simulink model "ReverseParking_Model"  (Simulink 8.2)
settings: Solver=FixedStepDiscrete  SolverMode=SingleTasking  StartTime=0.0  StopTime=inf  FixedStep=1/100  RelTol=1e-3
values from neighbouring files (symbols this model uses):
  dfreq = block.DialogPrm(1).Data    [msfcn_PPS_PlotSpeed.m]    (also in msfcn_PPS_radar_graph.m)
libraries: simulink x16, simulink_extras x3
settings Model: Creator=Krzysztof  LastModifiedBy=raufk
settings DataIOCC: SaveOutput=off  SaveTime=off
settings OptimizationCC: InlineParams=on  OptimizeBlockIOStorage=off  BufferReuse=off  ExpressionFolding=off  LocalBlockOutputs=off  SimCompilerOptimization=On
settings DebuggingCC: ReadBeforeWriteMsg=DisableAll  WriteAfterWriteMsg=DisableAll  WriteAfterReadMsg=DisableAll  SolverPrmCheckMsg=none  MultiTaskDSMMsg=none  SigSpecEnsureSampleTimeMsg=none  ParameterPrecisionLossMsg=none  FrameProcessingCompatibilityMsg=error  UnknownTsInhSupMsg=none
settings ModelReferenceCC: ModelReferenceNumInstancesAllowed=Single
settings SFSimCC: SimParseCustomCode=off
settings GRTTargetCC: CodeReplacementLibrary=C89/C90 (ANSI)

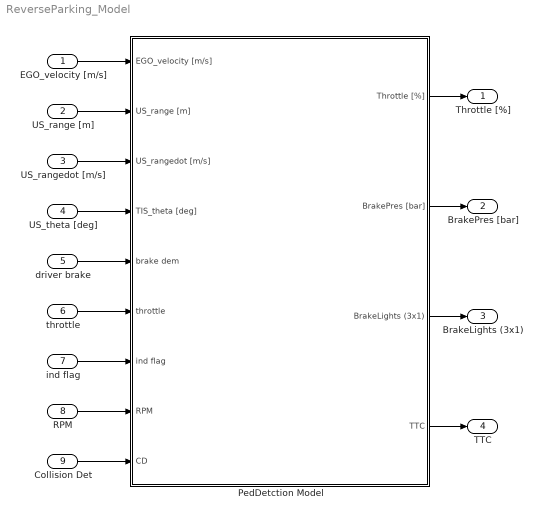
== system ReverseParking_Model ==
  EGO_velocity [m/s] : Inport
  US_range [m] : Inport  Port=2
  US_rangedot [m/s] : Inport  Port=3
  US_theta [deg] : Inport  Port=4
  driver brake : Inport  Port=5
  throttle : Inport  Port=6
  ind flag : Inport  Port=7
  RPM : Inport  Port=8
  Collision Det : Inport  Port=9
  PedDetction Model : Subsystem  mask(PPS Model){MaxSpeed=70, MaxBrakePressure=150, BrakeDelay=100, LaneWidth=3.5, USMaxRange=3, USMaxTheta=90, USfreq=20, USdet=2, Mainfreq=100}
      mask prompts: MaxSpeed "Vehicle cut-off speed [km/h]"; MaxBrakePressure "Maximum value of braking pressure available [bar]"; BrakeDelay "Braking system delay [ms]"; LaneWidth "Lane width [m]"; USMaxRange "US maximum range [m]"; USMaxTheta "US maximum theta [deg]"; USfreq "US frequency [Hz]"; USdet "Maximum Number of US Detected Objects"; Mainfreq "Compilation sheet frequency [Hz]"
      mask help: PreScan Experiment and Pedestrian Protection System parameters
      mask Help: eval('openHelp(8130)')
  Throttle [%] : Outport
  BrakePres [bar] : Outport  Port=2
  BrakeLights (3x1) : Outport  Port=3
  TTC : Outport  Port=4
  wires:
  EGO_velocity [m/s]/1 -> PedDetction Model/1(EGO_velocity [m/s])
  US_range [m]/1 -> PedDetction Model/2(US_range [m])
  US_rangedot [m/s]/1 -> PedDetction Model/3(US_rangedot [m/s])
  US_theta [deg]/1 -> PedDetction Model/4(TIS_theta [deg])
  throttle/1 -> PedDetction Model/6(throttle)
  ind flag/1 -> PedDetction Model/7(ind flag)
  PedDetction Model/1(Throttle [%]) -> Throttle [%]/1
  PedDetction Model/2(BrakePres [bar]) -> BrakePres [bar]/1
  PedDetction Model/3(BrakeLights (3x1)) -> BrakeLights (3x1)/1
  PedDetction Model/4(TTC) -> TTC/1
  driver brake/1 -> PedDetction Model/5(brake dem)
  RPM/1 -> PedDetction Model/8(RPM)
  Collision Det/1 -> PedDetction Model/9(CD)

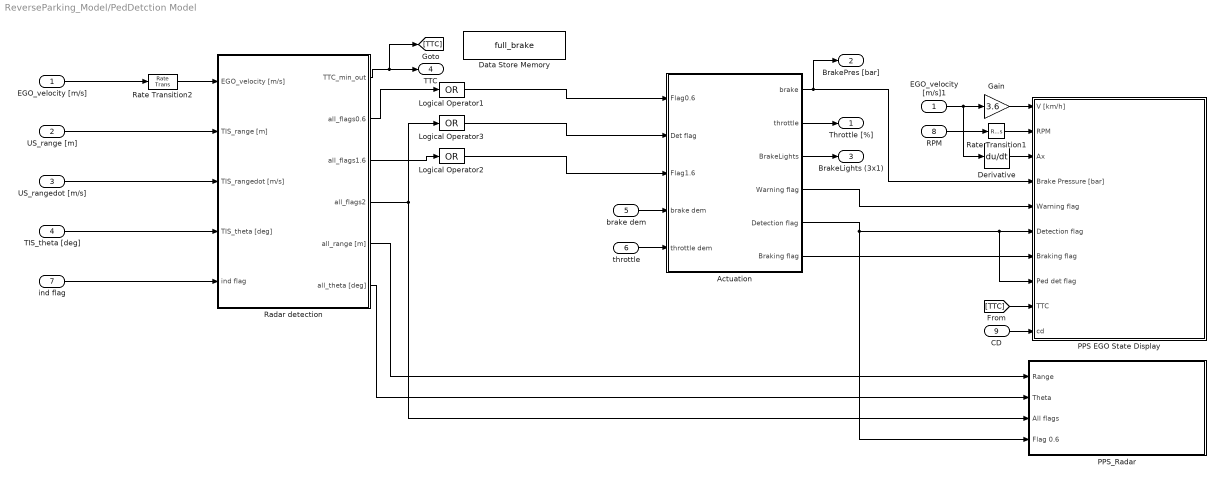
== system ReverseParking_Model/PedDetction Model ==
  EGO_velocity [m/s] : Inport
  US_range [m] : Inport  Port=2  PortDimensions=USdet  SampleTime=1/USfreq
  US_rangedot [m/s] : Inport  Port=3  PortDimensions=USdet  SampleTime=1/USfreq
  TIS_theta [deg] : Inport  Port=4  PortDimensions=USdet  SampleTime=1/USfreq
  brake dem : Inport  Port=5  SampleTime=[0,0]
  throttle : Inport  Port=6  SampleTime=[0,0]
  ind flag : Inport  Port=7  SampleTime=1/USfreq
  RPM : Inport  Port=8
  CD : Inport  Port=9
  Actuation : Subsystem
  Data Store Memory : DataStoreMemory  DataStoreName=full_brake  ReadBeforeWriteMsg=warning  WriteAfterWriteMsg=warning  WriteAfterReadMsg=warning
  Derivative : Derivative
  EGO_velocity [m/s]1 : InportShadow
  Gain : Gain  Gain=3.6
  Logical Operator1 : Logic  Operator=OR  Inputs=1  AllPortsSameDT=off  OutDataTypeStr=boolean
  Logical Operator2 : Logic  Operator=OR  Inputs=1  AllPortsSameDT=off  OutDataTypeStr=boolean
  Logical Operator3 : Logic  Operator=OR  Inputs=1  AllPortsSameDT=off  OutDataTypeStr=boolean
  PPS EGO State Display : Subsystem  StopFcn=|
      | load('VRU_DisplaySwitch');
      | load('VRU_EGO_State_Coll');
      | load('VRU_EGO_State_BrakeVel');
      | load('VRU_EGO_State_Flag06');
      | s_VRU_DisplaySwitch = VRU_DisplaySwitch(2,end);
      | s_VRU_EGO_State_Coll = VRU_EGO_State_Coll(2,end);
      | s_VRU_EGO_State_BrakeVel = VRU_EGO_State_BrakeVel(2,end);
      | s_VRU_EGO_State_Flag06 = VRU_EGO_State_Flag06(2,end);
      | 
      | if(s_VRU_DisplaySwitch)
      |   CSpanel = findobj('Tag','cs_panel');
      |   CSvalue = findobj('Tag','cs_value');
      |   
      |   if(s_VRU_EGO_State_Coll)
      |      %Collision Occured
      |      set(CSpanel, 'BorderWidth',2, 'ForegroundColor',[0 120/255 0], 'HighlightColor',[0 120/255 0], 'ShadowColor', [0 120/255 0]);
      |      set(CSvalue, 'ForegroundColor',[0 120/255 0], 'String', strcat('Speed reduction', sprintf( ' %.1f ',s_VRU_EGO_State_BrakeVel-s_VRU_EGO_State_Coll), ' km/h'));
      |      set(CSpanel, 'Visible', 'On');
      |      set(CSvalue, 'Visible', 'On');
      |   else
      |     if(s_VRU_EGO_State_Flag06)
      |         % Collision almost occur
      |         set(CSpanel, 'BorderWidth',2, 'ForegroundColor','Green', 'HighlightColor','Green', 'ShadowColor', 'Green');
      |         set(CSvalue, 'ForegroundColor','Green', 'String', 'Collision avoided');
      |         set(CSpanel, 'Visible', 'On');
      |         set(CSvalue, 'Visible', 'On');
      |      else
      |         % No risk of collision
      |         set(CSpanel, 'Visible', 'Off');
      |         set(CSvalue, 'Visible', 'Off');
      |     end
      |   end
      | 
      |   clear CSpanel CSvalue
      | end
      | 
      | PPS_Speed_Profile
      | PPS_TTC_Profile
  PPS_Radar : Subsystem
  Radar detection : Subsystem
  Rate Transition1 : RateTransition  Integrity=off  Deterministic=off  OutPortSampleTime=1/Mainfreq
  Rate Transition2 : RateTransition  Integrity=off  Deterministic=off  OutPortSampleTime=1/USfreq
  Throttle [%] : Outport
  BrakePres [bar] : Outport  Port=2
  BrakeLights (3x1) : Outport  Port=3
  TTC : Outport  Port=4
  wires:
  US_range [m]/1 -> Radar detection/2(TIS_range [m])
  US_rangedot [m/s]/1 -> Radar detection/3(TIS_rangedot [m/s])
  TIS_theta [deg]/1 -> Radar detection/4(TIS_theta [deg])
  ind flag/1 -> Radar detection/5(ind flag)
  EGO_velocity [m/s]/1 -> Rate Transition2/1
  Rate Transition2/1 -> Radar detection/1(EGO_velocity [m/s])
  throttle/1 -> Actuation/5(throttle dem)
  brake dem/1 -> Actuation/4(brake dem)
  Radar detection/1(TTC_min_out) -> TTC/1, [TTC]
  Radar detection/2(all_flags0.6) -> Logical Operator1/1
  Radar detection/4(all_flags2) -> PPS_Radar/3(All flags), Logical Operator3/1
  Radar detection/5(all_range [m]) -> PPS_Radar/1(Range)
  Radar detection/6(all_theta [deg]) -> PPS_Radar/2(Theta)
  Radar detection/3(all_flags1.6) -> Logical Operator2/1
  Actuation/1(brake) -> BrakePres [bar]/1, PPS EGO State Display/4(Brake Pressure [bar])
  Actuation/2(throttle) -> Throttle [%]/1
  Actuation/3(BrakeLights) -> BrakeLights (3x1)/1
  Actuation/6(Braking flag) -> PPS EGO State Display/7(Braking flag)
  Logical Operator1/1 -> Actuation/1(Flag0.6)
  Logical Operator2/1 -> Actuation/3(Flag1.6)
  Logical Operator3/1 -> Actuation/2(Det flag)
  EGO_velocity [m/s]1/1 -> Gain/1, Derivative/1
  Gain/1 -> PPS EGO State Display/1(V [km/h])
  RPM/1 -> Rate Transition1/1
  Derivative/1 -> PPS EGO State Display/3(Ax)
  CD/1 -> PPS EGO State Display/10(cd)
  [TTC] -> PPS EGO State Display/9(TTC)
  Actuation/4(Warning flag) -> PPS EGO State Display/5(Warning flag)
  Actuation/5(Detection flag) -> PPS_Radar/4(Flag 0.6), PPS EGO State Display/8(Ped det flag), PPS EGO State Display/6(Detection flag)
  Rate Transition1/1 -> PPS EGO State Display/2(RPM)

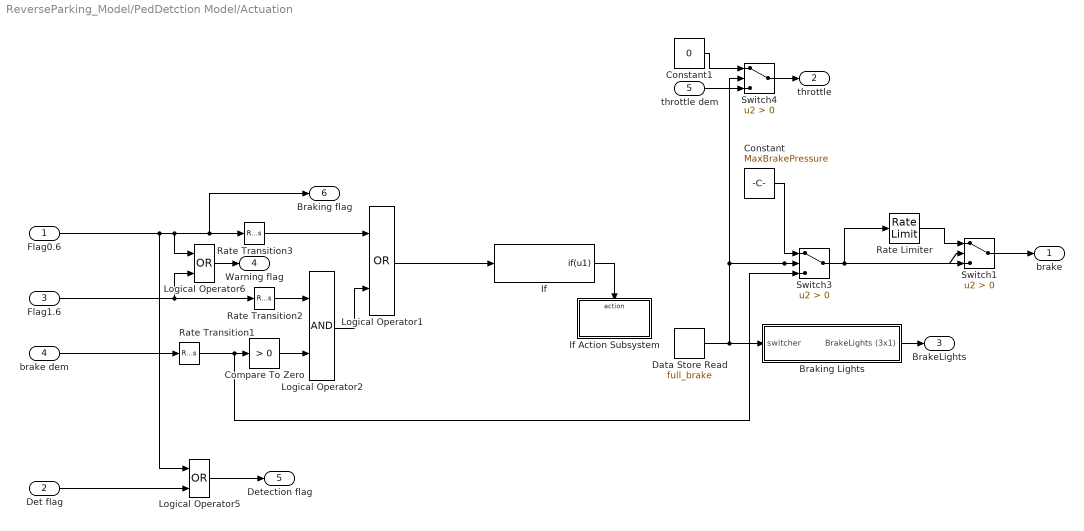
== system ReverseParking_Model/PedDetction Model/Actuation ==
  Flag0.6 : Inport
  Det flag : Inport  Port=2
  Flag1.6 : Inport  Port=3
  brake dem : Inport  Port=4
  throttle dem : Inport  Port=5
  Braking Lights : Subsystem
  Compare To Zero : simulink/Logic and Bit Operations/Compare To Zero  relop=>  OutDataTypeStr=uint8
  Constant : Constant  Value=MaxBrakePressure  SampleTime=[0,0]
  Constant1 : Constant  Value=0  SampleTime=[0,0]
  Data Store Read : DataStoreRead  DataStoreName=full_brake  SampleTime=1/Mainfreq
  If : If  IfExpression=u1  ShowElse=off
  If Action Subsystem : Subsystem  TreatAsAtomicUnit=on
  Logical Operator1 : Logic  Operator=OR  AllPortsSameDT=off  OutDataTypeStr=boolean  SampleTime=[0,0]
  Logical Operator2 : Logic  AllPortsSameDT=off  OutDataTypeStr=boolean  SampleTime=[0,0]
  Logical Operator5 : Logic  Operator=OR  AllPortsSameDT=off  OutDataTypeStr=boolean  SampleTime=1/USfreq
  Logical Operator6 : Logic  Operator=OR  AllPortsSameDT=off  OutDataTypeStr=boolean  SampleTime=1/USfreq
  Rate Limiter : RateLimiter  RisingSlewLimit=1000*0.9*MaxBrakePressure/BrakeDelay  FallingSlewLimit=-inf  SampleTimeMode=inherited
  Rate Transition1 : RateTransition  Integrity=off  OutPortSampleTime=[0,0]
  Rate Transition2 : RateTransition  Integrity=off  OutPortSampleTime=[0,0]
  Rate Transition3 : RateTransition  Integrity=off  OutPortSampleTime=[0,0]
  Switch1 : Switch  Criteria=u2 > Threshold  SampleTime=[0,0]
  Switch3 : Switch  Criteria=u2 > Threshold  SampleTime=[0,0]
  Switch4 : Switch  Criteria=u2 > Threshold  SampleTime=[0,0]
  brake : Outport  SampleTime=[0,0]
  throttle : Outport  Port=2  SampleTime=[0,0]
  BrakeLights : Outport  Port=3  SampleTime=1/Mainfreq
  Warning flag : Outport  Port=4
  Detection flag : Outport  Port=5
  Braking flag : Outport  Port=6
  wires:
  Logical Operator2/1 -> Logical Operator1/2
  Compare To Zero/1 -> Logical Operator2/2
  Constant/1 -> Switch3/1
  Constant1/1 -> Switch4/1
  Switch4/1 -> throttle/1
  throttle dem/1 -> Switch4/3
  Braking Lights/1(BrakeLights (3x1)) -> BrakeLights/1
  brake dem/1 -> Rate Transition1/1
  Rate Transition1/1 -> Compare To Zero/1, Switch3/3
  Rate Transition2/1 -> Logical Operator2/1
  Rate Transition3/1 -> Logical Operator1/1
  Switch3/1 -> Switch1/3, Rate Limiter/1
  Rate Limiter/1 -> Switch1/1
  Switch1/1 -> brake/1
  Flag0.6/1 -> Logical Operator5/1, Rate Transition3/1, Braking flag/1, Logical Operator6/1
  Flag1.6/1 -> Rate Transition2/1, Logical Operator6/2
  Logical Operator6/1 -> Warning flag/1
  Det flag/1 -> Logical Operator5/2
  Logical Operator5/1 -> Detection flag/1
  Logical Operator1/1 -> If/1
  Data Store Read/1 -> Braking Lights/1(switcher), Switch4/2, Switch3/2, Switch1/2
  If/1 -> If Action Subsystem/Action

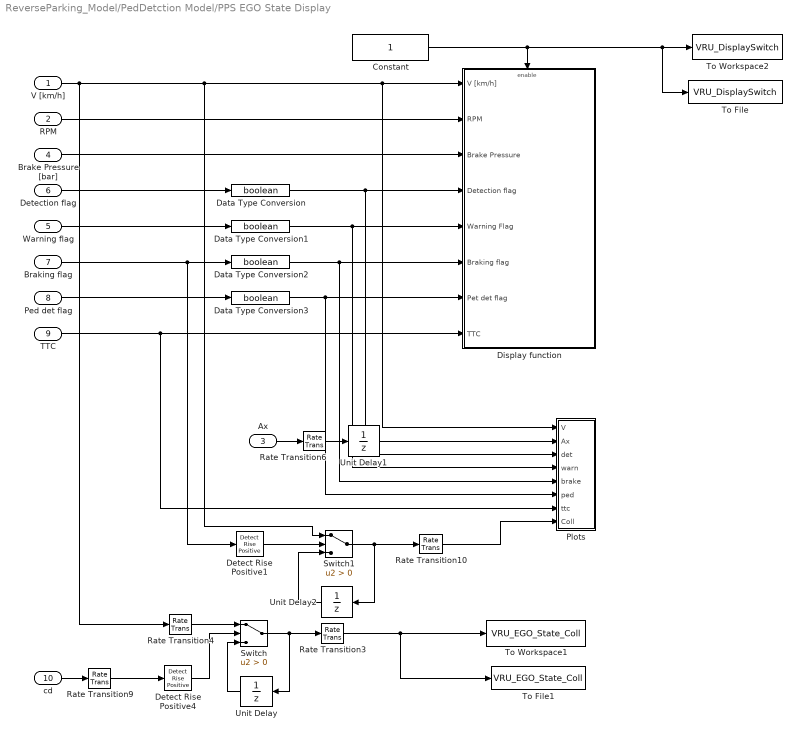
== system ReverseParking_Model/PedDetction Model/PPS EGO State Display ==
  V [km/h] : Inport
  RPM : Inport  Port=2
  Ax : Inport  Port=3  SampleTime=[0,0]
  Brake Pressure [bar] : Inport  Port=4
  Warning flag : Inport  Port=5  OutDataTypeStr=boolean
  Detection flag : Inport  Port=6  OutDataTypeStr=boolean
  Braking flag : Inport  Port=7  OutDataTypeStr=boolean
  Ped det flag : Inport  Port=8  OutDataTypeStr=boolean
  TTC : Inport  Port=9
  cd : Inport  Port=10  OutDataTypeStr=boolean
  Constant : Constant
  Data Type Conversion{,1..3} (4 alike) : DataTypeConversion  OutDataTypeStr=boolean
  Detect Rise Positive1 : simulink/Logic and Bit Operations/Detect Rise Positive  vinit=0  InputProcessing=Inherited  OutDataTypeStr=uint8
  Detect Rise Positive4 : simulink/Logic and Bit Operations/Detect Rise Positive  vinit=0  InputProcessing=Inherited  OutDataTypeStr=uint8
  Display function : Subsystem
  Plots : Subsystem
      mask help:
      | The block calls functions:
      | * PPS_Speed_Profile
      | * PPS_TTC_Profile
      | to generate plots at the end of the simulation.
      | See stop callback of the block for more details.
  Rate Transition10 : RateTransition  Integrity=off  OutPortSampleTime=[0,0]
  Rate Transition3 : RateTransition  Integrity=off  OutPortSampleTime=[0,0]
  Rate Transition4 : RateTransition  Integrity=off  OutPortSampleTime=1/Mainfreq
  Rate Transition6 : RateTransition  Integrity=off  OutPortSampleTimeOpt=Inherit  OutPortSampleTime=1/dfreq
  Rate Transition9 : RateTransition  Integrity=off  OutPortSampleTime=1/Mainfreq
  Switch : Switch  Criteria=u2 > Threshold  SampleTime=1/Mainfreq
  Switch1 : Switch  Criteria=u2 > Threshold  SampleTime=1/Mainfreq
  To File : ToFile  Filename=VRU_DisplaySwitch  MatrixName=VRU_DisplaySwitch  SampleTime=1/Mainfreq
  To File1 : ToFile  Filename=VRU_EGO_State_Coll  MatrixName=VRU_EGO_State_Coll  SampleTime=1/Mainfreq
  To Workspace1 : ToWorkspace  VariableName=VRU_EGO_State_Coll  SampleTime=1/Mainfreq
      settings: MaxDataPoints=1
  To Workspace2 : ToWorkspace  VariableName=VRU_DisplaySwitch  SampleTime=1/Mainfreq
      settings: MaxDataPoints=1
  Unit Delay : UnitDelay  SampleTime=1/Mainfreq
  Unit Delay1 : UnitDelay  SampleTime=-1
  Unit Delay2 : UnitDelay  SampleTime=1/Mainfreq
  wires:
  Warning flag/1 -> Data Type Conversion1/1
  Ped det flag/1 -> Data Type Conversion3/1
  Detection flag/1 -> Data Type Conversion/1
  V [km/h]/1 -> Display function/1(V [km/h]), Plots/1(V), Switch1/1, Rate Transition4/1
  RPM/1 -> Display function/2(RPM)
  Rate Transition3/1 -> To File1/1, To Workspace1/1
  cd/1 -> Rate Transition9/1
  Switch/1 -> Unit Delay/1, Rate Transition3/1
  Unit Delay/1 -> Switch/3
  Rate Transition4/1 -> Switch/1
  Detect Rise Positive4/1 -> Switch/2
  Braking flag/1 -> Data Type Conversion2/1, Detect Rise Positive1/1
  Ax/1 -> Rate Transition6/1
  Rate Transition6/1 -> Unit Delay1/1
  Brake Pressure [bar]/1 -> Display function/3(Brake Pressure)
  Unit Delay1/1 -> Plots/2(Ax)
  TTC/1 -> Plots/7(ttc), Display function/8(TTC)
  Rate Transition9/1 -> Detect Rise Positive4/1
  Data Type Conversion3/1 -> Plots/6(ped), Display function/7(Pet det flag)
  Data Type Conversion2/1 -> Display function/6(Braking flag), Plots/5(brake)
  Data Type Conversion1/1 -> Plots/4(warn), Display function/5(Warning Flag)
  Data Type Conversion/1 -> Plots/3(det), Display function/4(Detection flag)
  Constant/1 -> Display function/Enable, To File/1, To Workspace2/1
  Detect Rise Positive1/1 -> Switch1/2
  Switch1/1 -> Unit Delay2/1, Rate Transition10/1
  Unit Delay2/1 -> Switch1/3
  Rate Transition10/1 -> Plots/8(Coll)

== system ReverseParking_Model/PedDetction Model/PPS_Radar ==
  Range : Inport
  Theta : Inport  Port=2
  All flags : Inport  Port=3  OutDataTypeStr=boolean
  Flag 0.6 : Inport  Port=4  OutDataTypeStr=boolean
  Constant : Constant
  Radar : Subsystem
  wires:
  Range/1 -> Radar/1(Range)
  Theta/1 -> Radar/2(Theta)
  All flags/1 -> Radar/3(All flags)
  Flag 0.6/1 -> Radar/4(Flag 0.6)
  Constant/1 -> Radar/Enable

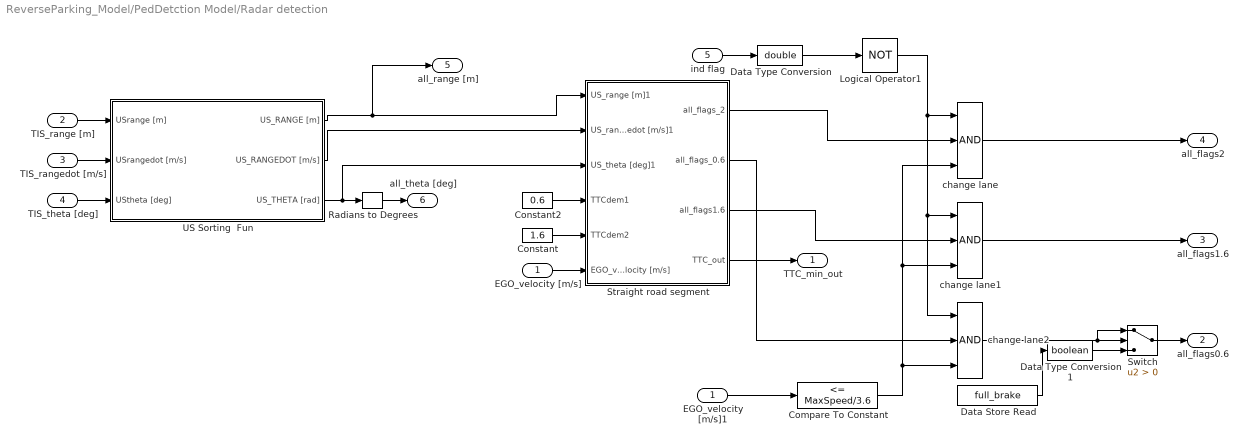
== system ReverseParking_Model/PedDetction Model/Radar detection ==
  EGO_velocity [m/s] : Inport
  TIS_range [m] : Inport  Port=2  PortDimensions=USdet
  TIS_rangedot [m/s] : Inport  Port=3  PortDimensions=USdet
  TIS_theta [deg] : Inport  Port=4  PortDimensions=USdet
  ind flag : Inport  Port=5
  Compare To Constant : simulink/Logic and Bit Operations/Compare To Constant  relop=<=  const=MaxSpeed/3.6  OutDataTypeStr=uint8
  Constant : Constant  Value=1.6
  Constant2 : Constant  Value=0.6
  Data Store Read : DataStoreRead  DataStoreName=full_brake  SampleTime=1/Mainfreq
  Data Type Conversion : DataTypeConversion  OutDataTypeStr=double
  Data Type Conversion1 : DataTypeConversion  OutDataTypeStr=boolean
  EGO_velocity [m/s]1 : InportShadow
  Logical Operator1 : Logic  Operator=NOT  AllPortsSameDT=off  OutDataTypeStr=boolean
  Radians to Degrees : simulink_extras/Transformations/Radians to Degrees
  Straight road segment : Subsystem  TreatAsAtomicUnit=on
  Switch : Switch  Criteria=u2 > Threshold
  US Sorting  Fun : Subsystem
  change lane : Logic  Inputs=3  AllPortsSameDT=off  OutDataTypeStr=boolean
  change lane1 : Logic  Inputs=3  AllPortsSameDT=off  OutDataTypeStr=boolean
  change lane2 : Logic  Inputs=3  AllPortsSameDT=off  OutDataTypeStr=boolean
  TTC_min_out : Outport
  all_flags0.6 : Outport  Port=2
  all_flags1.6 : Outport  Port=3
  all_flags2 : Outport  Port=4
  all_range [m] : Outport  Port=5
  all_theta [deg] : Outport  Port=6
  wires:
  TIS_range [m]/1 -> US Sorting  Fun/1(USrange [m])
  TIS_rangedot [m/s]/1 -> US Sorting  Fun/2(USrangedot [m/s])
  TIS_theta [deg]/1 -> US Sorting  Fun/3(UStheta [deg])
  US Sorting  Fun/1(US_RANGE [m]) -> Straight road segment/1(US_range [m]1), all_range [m]/1
  US Sorting  Fun/2(US_RANGEDOT [m/s]) -> Straight road segment/2(US_rangedot [m/s]1)
  US Sorting  Fun/3(US_THETA [rad]) -> Straight road segment/3(US_theta [deg]1), Radians to Degrees/1
  Constant2/1 -> Straight road segment/4(TTCdem1)
  Constant/1 -> Straight road segment/5(TTCdem2)
  EGO_velocity [m/s]/1 -> Straight road segment/6(EGO_velocity [m/s])
  ind flag/1 -> Data Type Conversion/1
  Radians to Degrees/1 -> all_theta [deg]/1
  Data Type Conversion/1 -> Logical Operator1/1
  Straight road segment/4(TTC_out) -> TTC_min_out/1
  Straight road segment/1(all_flags_2) -> change lane/2
  Logical Operator1/1 -> change lane/1, change lane2/1, change lane1/1
  Straight road segment/3(all_flags1.6) -> change lane1/2
  Straight road segment/2(all_flags_0.6) -> change lane2/2
  change lane/1 -> all_flags2/1
  Switch/1 -> all_flags0.6/1
  EGO_velocity [m/s]1/1 -> Compare To Constant/1
  Compare To Constant/1 -> change lane2/3, change lane1/3, change lane/3
  change lane1/1 -> all_flags1.6/1
  Data Store Read/1 -> Data Type Conversion1/1
  change lane2/1 -> Switch/2, Switch/1
  Data Type Conversion1/1 -> Switch/3

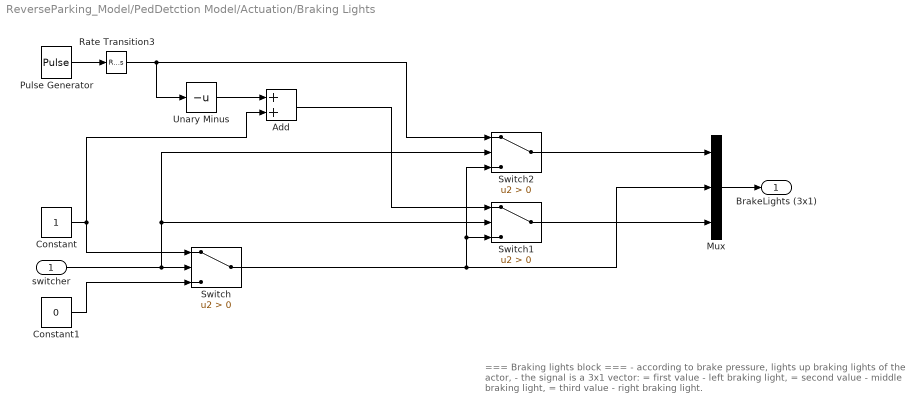
== system ReverseParking_Model/PedDetction Model/Actuation/Braking Lights ==
  note: === Braking lights block ===
      |
      |    - according to brake pressure, lights up braking lights of the actor,
      |    - the signal is a 3x1 vector:
      |      = first        value - left braking light,
      |      = second value - middle braking light,
      |      = third       value - right braking light.
  switcher : Inport
  Add : Sum
  Constant : Constant
  Constant1 : Constant  Value=0
  Mux : Mux  Inputs=3
  Pulse Generator : DiscretePulseGenerator  PulseType=Time based  Period=0.6  PulseWidth=50  PhaseDelay=0.3
  Rate Transition3 : RateTransition  Integrity=off  Deterministic=off  OutPortSampleTime=[0,0]
  Switch : Switch  Criteria=u2 > Threshold
  Switch1 : Switch  Criteria=u2 > Threshold
  Switch2 : Switch  Criteria=u2 > Threshold
  Unary Minus : UnaryMinus
  BrakeLights (3x1) : Outport
  wires:
  Mux/1 -> BrakeLights (3x1)/1
  switcher/1 -> Switch/2, Switch1/2, Switch2/2
  Constant/1 -> Switch/1, Add/2
  Switch/1 -> Switch1/3, Switch2/3, Mux/2
  Constant1/1 -> Switch/3
  Switch2/1 -> Mux/1
  Switch1/1 -> Mux/3
  Pulse Generator/1 -> Rate Transition3/1
  Add/1 -> Switch1/1
  Unary Minus/1 -> Add/1
  Rate Transition3/1 -> Unary Minus/1, Switch2/1

== system ReverseParking_Model/PedDetction Model/Actuation/If Action Subsystem ==
  Action Port : ActionPort  ActionType=then
  Constant1 : Constant  SampleTime=[0,0]
  Data Store Write : DataStoreWrite  DataStoreName=full_brake
  wires:
  Constant1/1 -> Data Store Write/1

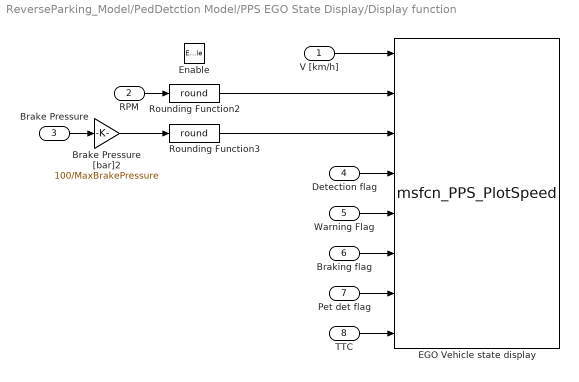
== system ReverseParking_Model/PedDetction Model/PPS EGO State Display/Display function ==
  V [km/h] : Inport
  RPM : Inport  Port=2
  Brake Pressure : Inport  Port=3
  Detection flag : Inport  Port=4
  Warning Flag : Inport  Port=5
  Braking flag : Inport  Port=6
  Pet det flag : Inport  Port=7
  TTC : Inport  Port=8
  Enable : EnablePort
  Brake Pressure [bar]2 : Gain  Gain=100/MaxBrakePressure
  EGO Vehicle state display : M-S-Function  FunctionName=msfcn_PPS_PlotSpeed  Parameters=USfreq 1
  Rounding Function2 : Rounding  Operator=round
  Rounding Function3 : Rounding  Operator=round
  wires:
  Brake Pressure [bar]2/1 -> Rounding Function3/1
  Rounding Function3/1 -> EGO Vehicle state display/3
  Rounding Function2/1 -> EGO Vehicle state display/2
  V [km/h]/1 -> EGO Vehicle state display/1
  Detection flag/1 -> EGO Vehicle state display/4
  Warning Flag/1 -> EGO Vehicle state display/5
  Braking flag/1 -> EGO Vehicle state display/6
  Pet det flag/1 -> EGO Vehicle state display/7
  TTC/1 -> EGO Vehicle state display/8
  RPM/1 -> Rounding Function2/1
  Brake Pressure/1 -> Brake Pressure [bar]2/1

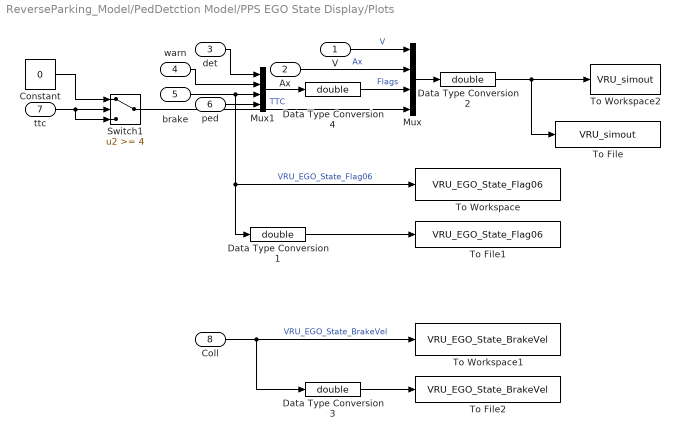
== system ReverseParking_Model/PedDetction Model/PPS EGO State Display/Plots ==
  V : Inport
  Ax : Inport  Port=2  SampleTime=[0,0]
  det : Inport  Port=3
  warn : Inport  Port=4
  brake : Inport  Port=5
  ped : Inport  Port=6
  ttc : Inport  Port=7
  Coll : Inport  Port=8
  Constant : Constant  Value=0
  Data Type Conversion{1..4} (4 alike) : DataTypeConversion  OutDataTypeStr=double
  Mux : Mux
  Mux1 : Mux
  Switch1 : Switch  Threshold=4
  To File : ToFile  Filename=VRU_simout  MatrixName=VRU_simout  SampleTime=1/Mainfreq
  To File1 : ToFile  Filename=VRU_EGO_State_Flag06  MatrixName=VRU_EGO_State_Flag06  SampleTime=1/Mainfreq
  To File2 : ToFile  Filename=VRU_EGO_State_BrakeVel  MatrixName=VRU_EGO_State_BrakeVel  SampleTime=1/Mainfreq
  To Workspace : ToWorkspace  VariableName=VRU_EGO_State_Flag06  SampleTime=-1
      settings: MaxDataPoints=1
  To Workspace1 : ToWorkspace  VariableName=VRU_EGO_State_BrakeVel  SampleTime=1/Mainfreq
      settings: MaxDataPoints=1
  To Workspace2 : ToWorkspace  VariableName=VRU_simout  SaveFormat=Structure With Time  SampleTime=0.04
  wires:
  Mux/1 -> Data Type Conversion2/1
  Mux1/1 -> Data Type Conversion4/1
  Data Type Conversion4/1 -> Mux/3  "Flags"
  Ax/1 -> Mux/2  "Ax"
  Switch1/1 -> Mux/4  "TTC"
  Constant/1 -> Switch1/1
  V/1 -> Mux/1  "V"
  det/1 -> Mux1/1
  warn/1 -> Mux1/2
  brake/1 -> Mux1/3, Data Type Conversion1/1, To Workspace/1  "VRU_EGO_State_Flag06"
  ped/1 -> Mux1/4
  ttc/1 -> Switch1/2, Switch1/3
  Coll/1 -> Data Type Conversion3/1, To Workspace1/1  "VRU_EGO_State_BrakeVel"
  Data Type Conversion1/1 -> To File1/1
  Data Type Conversion2/1 -> To File/1, To Workspace2/1
  Data Type Conversion3/1 -> To File2/1

== system ReverseParking_Model/PedDetction Model/PPS_Radar/Radar ==
  Range : Inport
  Theta : Inport  Port=2
  All flags : Inport  Port=3
  Flag 0.6 : Inport  Port=4
  Enable : EnablePort
  DISPLAY1 : M-S-Function  FunctionName=msfcn_PPS_radar_graph  Parameters=USfreq USdet 1 USMaxRange USMaxTheta*pi/180
  Degrees to Radians : simulink_extras/Transformations/Degrees to Radians
  wires:
  Range/1 -> DISPLAY1/1
  Theta/1 -> Degrees to Radians/1
  All flags/1 -> DISPLAY1/3
  Flag 0.6/1 -> DISPLAY1/4
  Degrees to Radians/1 -> DISPLAY1/2

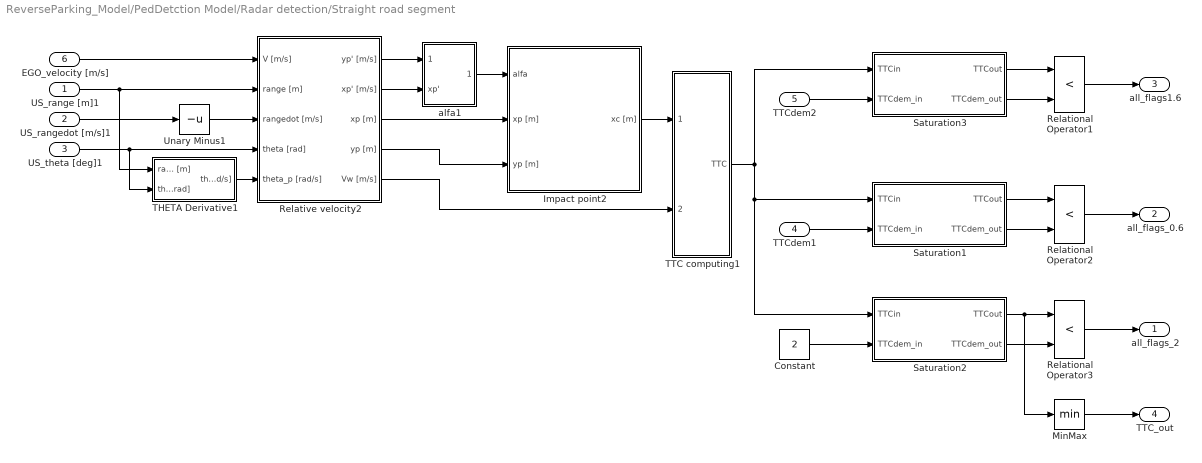
== system ReverseParking_Model/PedDetction Model/Radar detection/Straight road segment ==
  US_range [m]1 : Inport  PortDimensions=USdet
  US_rangedot [m/s]1 : Inport  Port=2  PortDimensions=USdet
  US_theta [deg]1 : Inport  Port=3  PortDimensions=USdet
  TTCdem1 : Inport  Port=4
  TTCdem2 : Inport  Port=5
  EGO_velocity [m/s] : Inport  Port=6
  Constant : Constant  Value=2
  Impact point2 : Subsystem
  MinMax : MinMax
  Relational Operator1 : RelationalOperator  Operator=<  OutDataTypeStr=fixdt(1,16)
  Relational Operator2 : RelationalOperator  Operator=<  OutDataTypeStr=fixdt(1,16)
  Relational Operator3 : RelationalOperator  Operator=<  OutDataTypeStr=fixdt(1,16)
  Relative velocity2 : Subsystem
  Saturation1 : Subsystem
  Saturation2 : Subsystem
  Saturation3 : Subsystem
  THETA Derivative1 : Subsystem
  TTC computing1 : Subsystem
  Unary Minus1 : UnaryMinus
  alfa1 : Subsystem
  all_flags_2 : Outport  InitialOutput=0
  all_flags_0.6 : Outport  Port=2  SampleTime=1/USfreq  InitialOutput=0
  all_flags1.6 : Outport  Port=3  SampleTime=1/USfreq  InitialOutput=0
  TTC_out : Outport  Port=4
  wires:
  EGO_velocity [m/s]/1 -> Relative velocity2/1(V [m/s])
  US_range [m]1/1 -> THETA Derivative1/1(range [m]), Relative velocity2/2(range [m])
  US_rangedot [m/s]1/1 -> Unary Minus1/1
  US_theta [deg]1/1 -> Relative velocity2/4(theta [rad]), THETA Derivative1/2(theta [rad])
  THETA Derivative1/1(theta_dot [rad/s]) -> Relative velocity2/5(theta_p [rad/s])
  Relative velocity2/1(yp' [m/s]) -> alfa1/1(yp'1)
  Relative velocity2/2(xp' [m/s]) -> alfa1/2(xp')
  Relative velocity2/3(xp [m]) -> Impact point2/2(xp [m])
  alfa1/1(alfa1) -> Impact point2/1(alfa)
  Unary Minus1/1 -> Relative velocity2/3(rangedot [m/s])
  Relative velocity2/4(yp [m]) -> Impact point2/3(yp [m])
  Impact point2/1(xc [m]) -> TTC computing1/1(xc [m])
  Relative velocity2/5(Vw [m/s]) -> TTC computing1/2(Vw [m/s])
  TTC computing1/1(TTC) -> Saturation1/1(TTCin), Saturation2/1(TTCin), Saturation3/1(TTCin)
  Saturation3/1(TTCout) -> Relational Operator1/1
  Relational Operator1/1 -> all_flags1.6/1
  TTCdem2/1 -> Saturation3/2(TTCdem_in)
  Saturation3/2(TTCdem_out) -> Relational Operator1/2
  Relational Operator2/1 -> all_flags_0.6/1
  TTCdem1/1 -> Saturation1/2(TTCdem_in)
  Saturation1/1(TTCout) -> Relational Operator2/1
  Saturation1/2(TTCdem_out) -> Relational Operator2/2
  Constant/1 -> Saturation2/2(TTCdem_in)
  Saturation2/2(TTCdem_out) -> Relational Operator3/2
  Saturation2/1(TTCout) -> Relational Operator3/1, MinMax/1
  Relational Operator3/1 -> all_flags_2/1
  MinMax/1 -> TTC_out/1

== system ReverseParking_Model/PedDetction Model/Radar detection/US Sorting  Fun ==
  USrange [m] : Inport
  USrangedot [m/s] : Inport  Port=2
  UStheta [deg] : Inport  Port=3
  Degrees to Radians : simulink_extras/Transformations/Degrees to Radians
  Switch : Switch  Criteria=u2 ~= 0
  Unary Minus : UnaryMinus
  Unary Minus1 : UnaryMinus
  range max : Constant  Value=USMaxRange
  US_RANGE [m] : Outport
  US_RANGEDOT [m/s] : Outport  Port=2
  US_THETA [rad] : Outport  Port=3
  wires:
  Unary Minus/1 -> Degrees to Radians/1
  Switch/1 -> US_RANGE [m]/1
  USrangedot [m/s]/1 -> Unary Minus1/1
  range max/1 -> Switch/3
  Degrees to Radians/1 -> US_THETA [rad]/1
  USrange [m]/1 -> Switch/1, Switch/2
  UStheta [deg]/1 -> Unary Minus/1
  Unary Minus1/1 -> US_RANGEDOT [m/s]/1

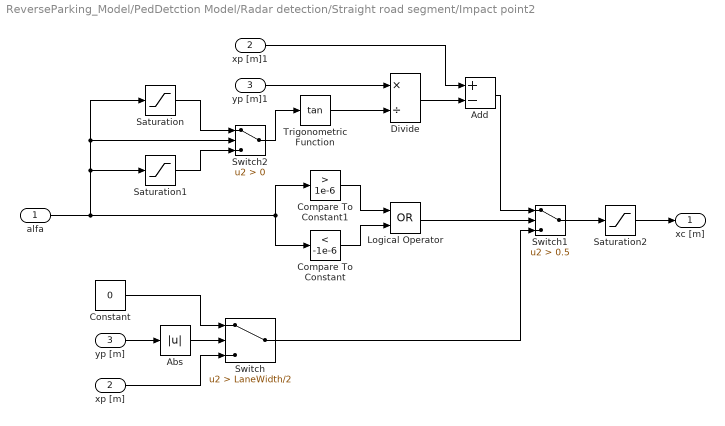
== system ReverseParking_Model/PedDetction Model/Radar detection/Straight road segment/Impact point2 ==
  alfa : Inport
  xp [m] : Inport  Port=2
  yp [m] : Inport  Port=3
  Abs : Abs
  Add : Sum  Inputs=+-
  Compare To Constant : simulink/Logic and Bit Operations/Compare To Constant  relop=<  const=-1e-6  OutDataTypeStr=uint8  ZeroCross=off
  Compare To Constant1 : simulink/Logic and Bit Operations/Compare To Constant  relop=>  const=1e-6  OutDataTypeStr=uint8  ZeroCross=off
  Constant : Constant  Value=0
  Divide : Product  Inputs=*/
  Logical Operator : Logic  Operator=OR  AllPortsSameDT=off  OutDataTypeStr=boolean
  Saturation : Saturate  UpperLimit=inf  LowerLimit=1e-6
  Saturation1 : Saturate  UpperLimit=-1e-6  LowerLimit=-inf
  Saturation2 : Saturate  UpperLimit=300  LowerLimit=0
  Switch : Switch  Criteria=u2 > Threshold  Threshold=LaneWidth/2
  Switch1 : Switch  Criteria=u2 > Threshold  Threshold=0.5
  Switch2 : Switch  Criteria=u2 > Threshold
  Trigonometric Function : Trigonometry  Operator=tan
  xp [m]1 : InportShadow  Port=2
  yp [m]1 : InportShadow  Port=3
  xc [m] : Outport
  wires:
  yp [m]/1 -> Abs/1
  xp [m]/1 -> Switch/3
  Constant/1 -> Switch/1
  Switch/1 -> Switch1/3
  Abs/1 -> Switch/2
  xp [m]1/1 -> Add/1
  Divide/1 -> Add/2
  yp [m]1/1 -> Divide/1
  Trigonometric Function/1 -> Divide/2
  alfa/1 -> Compare To Constant1/1, Compare To Constant/1, Saturation1/1, Switch2/2, Saturation/1
  Compare To Constant1/1 -> Logical Operator/1
  Compare To Constant/1 -> Logical Operator/2
  Logical Operator/1 -> Switch1/2
  Switch1/1 -> Saturation2/1
  Add/1 -> Switch1/1
  Switch2/1 -> Trigonometric Function/1
  Saturation/1 -> Switch2/1
  Saturation1/1 -> Switch2/3
  Saturation2/1 -> xc [m]/1

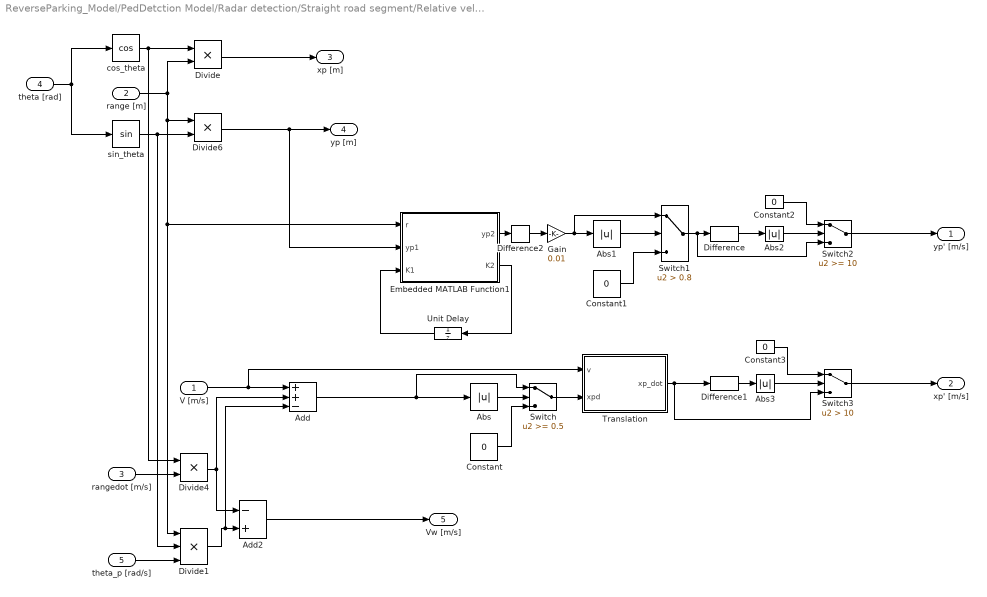
== system ReverseParking_Model/PedDetction Model/Radar detection/Straight road segment/Relative velocity2 ==
  V [m/s] : Inport
  range [m] : Inport  Port=2
  rangedot [m/s] : Inport  Port=3
  theta [rad] : Inport  Port=4
  theta_p [rad/s] : Inport  Port=5
  Abs{,1..3} (4 alike) : Abs
  Add : Sum  Inputs=++-
  Add2 : Sum  Inputs=-+
  Constant{,1..3} (4 alike) : Constant  Value=0
  Difference : simulink/Discrete/Difference  ICPrevInput=zeros(USdet,1)  InputProcessing=Inherited  OutMin=[]  OutMax=[]  OutDataType=fixdt(1, 16)  OutScaling=2^-10  DoSatur=off
  Difference1 : simulink/Discrete/Difference  ICPrevInput=zeros(USdet,1)  InputProcessing=Inherited  OutMin=[]  OutMax=[]  OutDataType=fixdt(1, 16)  OutScaling=2^-10  DoSatur=off
  Difference2 : simulink/Discrete/Difference  ICPrevInput=0.0  InputProcessing=Inherited  OutMin=[]  OutMax=[]  OutDataType=sfix(16)  OutScaling=2^-10  DoSatur=off
  Divide : Product  Inputs=**
  Divide1 : Product  Inputs=***
  Divide4 : Product  Inputs=**
  Divide6 : Product  Inputs=**
  Embedded MATLAB Function1 : MATLAB Function  TreatAsAtomicUnit=on  SystemSampleTime=0.01
      settings: PermitHierarchicalResolution=ParametersOnly
  Gain : Gain  Gain=0.01
  Switch : Switch  Threshold=0.5
  Switch1 : Switch  Criteria=u2 > Threshold  Threshold=0.8
  Switch2 : Switch  Threshold=10
  Switch3 : Switch  Criteria=u2 > Threshold  Threshold=10
  Translation : MATLAB Function  TreatAsAtomicUnit=on
      settings: PermitHierarchicalResolution=ParametersOnly
  Unit Delay : UnitDelay  InitialCondition=zeros(USdet,50)  SampleTime=-1
  cos_theta : Trigonometry  Operator=cos
  sin_theta : Trigonometry
  yp' [m/s] : Outport
  xp' [m/s] : Outport  Port=2
  xp [m] : Outport  Port=3
  yp [m] : Outport  Port=4
  Vw [m/s] : Outport  Port=5
  wires:
  rangedot [m/s]/1 -> Divide4/2
  Difference1/1 -> Abs3/1
  Constant3/1 -> Switch3/1
  Constant2/1 -> Switch2/1
  Switch3/1 -> xp' [m/s]/1
  Abs3/1 -> Switch3/2
  Translation/1(xp_dot) -> Difference1/1, Switch3/3
  Abs2/1 -> Switch2/2
  Difference/1 -> Abs2/1
  Switch2/1 -> yp' [m/s]/1
  Switch1/1 -> Switch2/3, Difference/1
  Constant1/1 -> Switch1/3
  Abs1/1 -> Switch1/2
  Gain/1 -> Switch1/1, Abs1/1
  Embedded MATLAB Function1/1(yp2) -> Difference2/1
  Unit Delay/1 -> Embedded MATLAB Function1/3(K1)
  Embedded MATLAB Function1/2(K2) -> Unit Delay/1
  Switch/1 -> Translation/2(xpd)
  Constant/1 -> Switch/3
  Abs/1 -> Switch/2
  Add/1 -> Switch/1, Abs/1
  V [m/s]/1 -> Translation/1(v), Add/1
  Divide1/1 -> Add/3, Add2/2
  Divide4/1 -> Add/2, Add2/1
  Add2/1 -> Vw [m/s]/1
  theta_p [rad/s]/1 -> Divide1/3
  Divide6/1 -> yp [m]/1, Embedded MATLAB Function1/2(yp1)
  cos_theta/1 -> Divide/1, Divide4/1
  sin_theta/1 -> Divide6/2, Divide1/2
  range [m]/1 -> Embedded MATLAB Function1/1(r), Divide1/1, Divide6/1, Divide/2
  Divide/1 -> xp [m]/1
  theta [rad]/1 -> cos_theta/1, sin_theta/1
  Difference2/1 -> Gain/1

== system ReverseParking_Model/PedDetction Model/Radar detection/Straight road segment/Saturation1 ==
  TTCin : Inport
  TTCdem_in : Inport  Port=2  SampleTime=1/USfreq
  Compare To Zero : simulink/Logic and Bit Operations/Compare To Zero  relop=<=  OutDataTypeStr=uint8
  Gain : Gain  Gain=2
  Gain1 : Gain  Gain=ones(USdet,1)
  Logical Operator : Logic  Operator=OR  AllPortsSameDT=off  OutDataTypeStr=boolean
  Relational Operator : RelationalOperator  Operator=>  OutDataTypeStr=boolean
  Switch : Switch  Criteria=u2 > Threshold  Threshold=0.5
  TTCout : Outport
  TTCdem_out : Outport  Port=2
  wires:
  Gain/1 -> Switch/1, Relational Operator/2
  Gain1/1 -> Gain/1, TTCdem_out/1
  Switch/1 -> TTCout/1
  TTCdem_in/1 -> Gain1/1
  Compare To Zero/1 -> Logical Operator/1
  Relational Operator/1 -> Logical Operator/2
  Logical Operator/1 -> Switch/2
  TTCin/1 -> Switch/3, Compare To Zero/1, Relational Operator/1

== system ReverseParking_Model/PedDetction Model/Radar detection/Straight road segment/Saturation2 ==
  TTCin : Inport
  TTCdem_in : Inport  Port=2  SampleTime=1/USfreq
  Compare To Zero : simulink/Logic and Bit Operations/Compare To Zero  relop=<=  OutDataTypeStr=uint8
  Gain : Gain  Gain=2
  Gain1 : Gain  Gain=ones(USdet,1)
  Logical Operator : Logic  Operator=OR  AllPortsSameDT=off  OutDataTypeStr=boolean
  Relational Operator : RelationalOperator  Operator=>  OutDataTypeStr=boolean
  Switch : Switch  Criteria=u2 > Threshold  Threshold=0.5
  TTCout : Outport
  TTCdem_out : Outport  Port=2
  wires:
  TTCin/1 -> Relational Operator/1, Compare To Zero/1, Switch/3
  Logical Operator/1 -> Switch/2
  Relational Operator/1 -> Logical Operator/2
  Compare To Zero/1 -> Logical Operator/1
  TTCdem_in/1 -> Gain1/1
  Switch/1 -> TTCout/1
  Gain1/1 -> TTCdem_out/1, Gain/1
  Gain/1 -> Relational Operator/2, Switch/1

== system ReverseParking_Model/PedDetction Model/Radar detection/Straight road segment/Saturation3 ==
  TTCin : Inport
  TTCdem_in : Inport  Port=2  SampleTime=1/USfreq
  Compare To Zero : simulink/Logic and Bit Operations/Compare To Zero  relop=<=  OutDataTypeStr=uint8
  Gain : Gain  Gain=2
  Gain1 : Gain  Gain=ones(USdet,1)
  Logical Operator : Logic  Operator=OR  AllPortsSameDT=off  OutDataTypeStr=boolean
  Relational Operator : RelationalOperator  Operator=>  OutDataTypeStr=boolean
  Switch : Switch  Criteria=u2 > Threshold  Threshold=0.5
  TTCout : Outport
  TTCdem_out : Outport  Port=2
  wires:
  TTCin/1 -> Relational Operator/1, Compare To Zero/1, Switch/3
  Logical Operator/1 -> Switch/2
  Relational Operator/1 -> Logical Operator/2
  Compare To Zero/1 -> Logical Operator/1
  TTCdem_in/1 -> Gain1/1
  Switch/1 -> TTCout/1
  Gain1/1 -> TTCdem_out/1, Gain/1
  Gain/1 -> Relational Operator/2, Switch/1

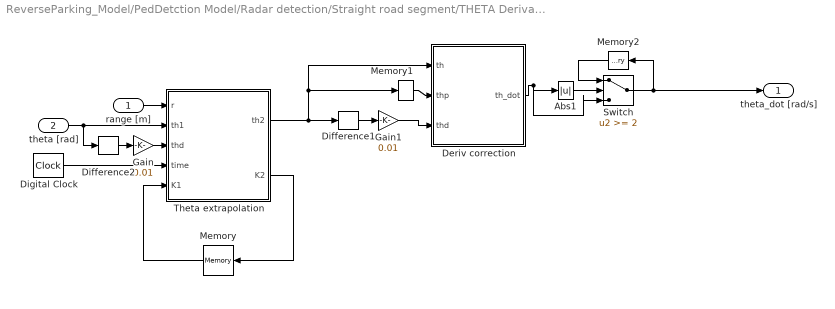
== system ReverseParking_Model/PedDetction Model/Radar detection/Straight road segment/THETA Derivative1 ==
  range [m] : Inport
  theta [rad] : Inport  Port=2
  Abs1 : Abs
  Deriv correction : MATLAB Function  TreatAsAtomicUnit=on
      settings: PermitHierarchicalResolution=ParametersOnly
  Difference1 : simulink/Discrete/Difference  ICPrevInput=0.0  InputProcessing=Inherited  OutMin=[]  OutMax=[]  OutDataType=sfix(16)  OutScaling=2^-10  DoSatur=off
  Difference2 : simulink/Discrete/Difference  ICPrevInput=0.0  InputProcessing=Inherited  OutMin=[]  OutMax=[]  OutDataType=sfix(16)  OutScaling=2^-10  DoSatur=off
  Digital Clock : DigitalClock  SampleTime=1/USfreq
  Gain : Gain  Gain=0.01
  Gain1 : Gain  Gain=0.01
  Memory : Memory  X0=zeros(USdet,10,2)  InheritSampleTime=on
  Memory1 : Memory  X0=zeros(USdet,1)  InheritSampleTime=on
  Memory2 : Memory  X0=zeros(USdet,1)  InheritSampleTime=on
  Switch : Switch  Threshold=2
  Theta extrapolation : MATLAB Function  TreatAsAtomicUnit=on
      settings: PermitHierarchicalResolution=ParametersOnly
  theta_dot [rad/s] : Outport
  wires:
  Memory1/1 -> Deriv correction/2(thp)
  Gain1/1 -> Deriv correction/3(thd)
  Theta extrapolation/1(th2) -> Deriv correction/1(th), Memory1/1, Difference1/1
  range [m]/1 -> Theta extrapolation/1(r)
  Gain/1 -> Theta extrapolation/3(thd)
  Digital Clock/1 -> Theta extrapolation/4(time)
  Memory/1 -> Theta extrapolation/5(K1)
  Theta extrapolation/2(K2) -> Memory/1
  theta [rad]/1 -> Theta extrapolation/2(th1), Difference2/1
  Deriv correction/1(th_dot) -> Switch/3, Abs1/1
  Switch/1 -> Memory2/1, theta_dot [rad/s]/1
  Abs1/1 -> Switch/2
  Memory2/1 -> Switch/1
  Difference2/1 -> Gain/1
  Difference1/1 -> Gain1/1

== system ReverseParking_Model/PedDetction Model/Radar detection/Straight road segment/TTC computing1 ==
  xc [m] : Inport
  Vw [m/s] : Inport  Port=2
  Compare To Constant : simulink/Logic and Bit Operations/Compare To Constant  relop===  const=1e-6  OutDataTypeStr=uint8  ZeroCross=off
  Constant : Constant  Value=0
  Data Type Conversion : DataTypeConversion  OutDataTypeStr=double
  Divide : Product  Inputs=/*
  Saturation : Saturate  UpperLimit=inf  LowerLimit=1e-6
  Switch : Switch  Criteria=u2 > Threshold
  Switch1 : Switch  Criteria=u2 > Threshold  Threshold=0.5
  TTC : Outport  InitialOutput=0
  wires:
  Vw [m/s]/1 -> Switch/2, Switch/1
  Constant/1 -> Switch/3, Switch1/1
  Switch/1 -> Saturation/1
  Saturation/1 -> Divide/1, Compare To Constant/1
  Compare To Constant/1 -> Data Type Conversion/1
  xc [m]/1 -> Divide/2
  Divide/1 -> Switch1/3
  Switch1/1 -> TTC/1
  Data Type Conversion/1 -> Switch1/2

== system ReverseParking_Model/PedDetction Model/Radar detection/Straight road segment/alfa1 ==
  yp'1 : Inport
  xp' : Inport  Port=2
  Abs : Abs
  Compare To Constant : simulink/Logic and Bit Operations/Compare To Constant  relop===  const=pi/2  OutDataTypeStr=uint8
  Constant : Constant  Value=0
  Switch : Switch  Criteria=u2 > Threshold
  four quadrant atan : Trigonometry  Operator=atan2
  alfa1 : Outport
  wires:
  yp'1/1 -> four quadrant atan/1
  xp'/1 -> four quadrant atan/2
  four quadrant atan/1 -> Abs/1, Switch/3
  Abs/1 -> Compare To Constant/1
  Compare To Constant/1 -> Switch/2
  Constant/1 -> Switch/1
  Switch/1 -> alfa1/1

== matlab function PedDetction Model/Radar detection/Straight road segment/Relative velocity2/Embedded MATLAB Function1 ==
  data: r input double; yp2 output double; yp1 input double; K1 input double; K2 output double; USdet parameter double; USMaxRange parameter double
function [yp2, K2] = modif(r, yp1, K1, USdet, USMaxRange)
%#eml
% Interpolating yp value.

K2 = K1;
yp2 = yp1;

d = 50;

% Adding point
for i = 1 : USdet
   if r(i) ~= 6
      K2(i,1:d-1) = K2(i,2:d);
      K2(i,d) = yp1(i);
   end
end

% Choosing what to take
for i = 1 : USdet
    s = 0;
    suma = 0;
    for j = 1 : 50
        if K2(i,j) ~= 0
            suma = suma + K2(i,j);
            s = s + 1;
        end
    end
    yp2(i) = suma/s;
end

% Returning, if object is not detected
for i = 1: USdet
    if r(i) == USMaxRange && yp1(i) == 0
        K2(i,:,:) = zeros(d,1);
        yp2(i) = 0;
    end    
end

== matlab function PedDetction Model/Radar detection/Straight road segment/Relative velocity2/Translation ==
  data: v input double; xpd input double; xp_dot output double; USdet parameter double
function xp_dot = trans(v, xpd, USdet)
%#codegen
%Translation of the value

xp_dot = xpd;
for i = 1 : USdet
    if xpd(i) == v
        xp_dot(i) =0;
    end
end
end

== matlab function PedDetction Model/Radar detection/Straight road segment/THETA Derivative1/Deriv correction ==
  data: th input double; thp input double; thd input double; th_dot output double; USdet parameter double
function th_dot = stopping(th, thp, thd, USdet)
%#codegen
% Stopping if nothing is detected.

th_dot = thd;
for i = 1 : USdet
    if (th(i)==0 && thp(i)~=0) || (th(i)~=0 && thp(i)==0)
        th_dot(i) = 0;
    end
end
end

== matlab function PedDetction Model/Radar detection/Straight road segment/THETA Derivative1/Theta extrapolation ==
  data: r input double; th1 input double; th2 output double; thd input double; time input double; K1 input double; K2 output double; USdet parameter double; USMaxRange parameter double
function [th2, K2] = modif(r, th1, thd, time, K1, USdet, USMaxRange)
%#codegen
% Interpolating theta value.

K2 = K1;
th2 = th1;

d = 10;

% Finding points used in interpolation/extrapolation.
for i = 1 : USdet
    if thd(i) ~= 0
        K2(i,1:d-1,:) = K2(i,2:d,:);
        K2(i,  d,1) = time;
        K2(i,  d,2) = th1(i);
    end
end

% Extrapolation
for i = 1 : USdet
    j = 1;
    while j < d+1 && K2(i,j,1) == 0
        j = j + 1;
    end
    
    if j > d-2
        th2(i) = th1(i);
    else
        th2(i) = interp1(K2(i,d-2:d,1),K2(i,d-2:d,2),time,'linear','extrap');
    end
end

% Returning, if object is not detected
for i = 1: USdet
    if r(i) == USMaxRange && th1(i) == 0
        K2(i,:,:) = zeros(d,2);
        th2(i) = 0;
    end    
end

end
